simulink model "damped_non_linear"  (R2019a)
settings: Solver=VariableStepAuto  StartTime=0.0  StopTime=10.0  RelTol=1e-3
settings Model: Creator=iyengar  LastModifiedBy=iyengar

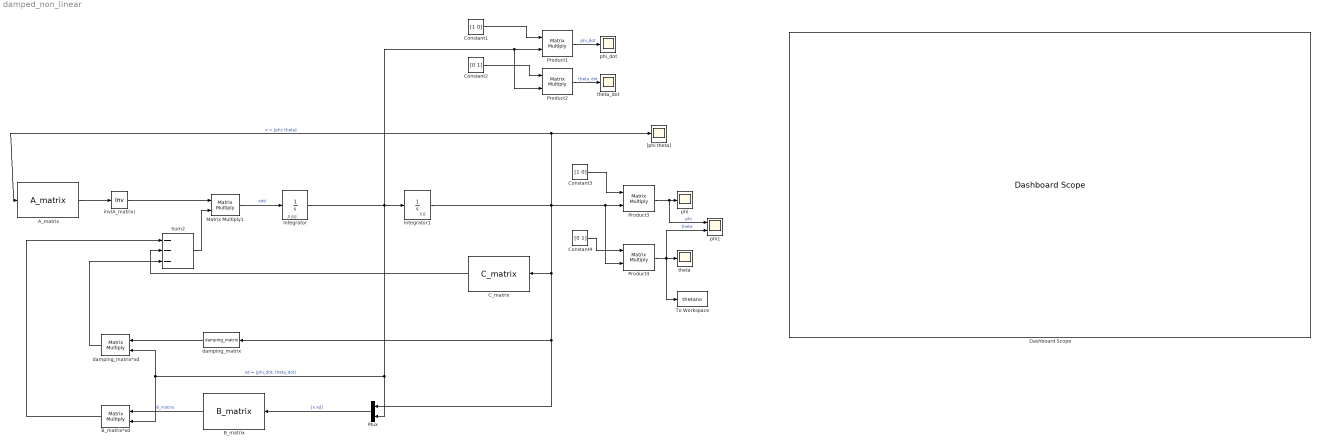
== system damped_non_linear ==
  note: Xdd
  note: Xd
  "A_matrix " : MATLABFcn  Description=matrix A. 2x2  MATLABFcn=A_matrix  OutputDimensions=[2, 2]  Output1D=off
  B_matrix : MATLABFcn  MATLABFcn=B_matrix  Output1D=off
  B_matrix*xd : Product  Multiplication=Matrix(*)
  C_matrix : MATLABFcn  MATLABFcn=C_matrix  OutputDimensions=2  Output1D=off
  Constant1 : Constant  Value=[1 0]  VectorParams1D=off
  Constant2 : Constant  Value=[0 1]  VectorParams1D=off
  Constant3 : Constant  Value=[1 0]  VectorParams1D=off
  Constant4 : Constant  Value=[0 1]  VectorParams1D=off
  Dashboard Scope : DashboardScope
  Integrator : Integrator  InitialCondition=[0; 0.5]
  Integrator1 : Integrator  InitialCondition=[0; 0.05]
  Matrix Multiply1 : Product  Multiplication=Matrix(*)
  Mux : Mux  Inputs=2
  Product{1..4} (4 alike) : Product  Multiplication=Matrix(*)
  Sum2 : Sum  Inputs=---
  To Workspace : ToWorkspace  VariableName=thetano  SaveFormat=Timeseries  SampleTime=-1
  "[phi theta]" : Scope
  damping_matrix : MATLABFcn  MATLABFcn=damping_matrix  Output1D=off
  "damping_matrix*xd " : Product  Multiplication=Matrix(*)
  inv(A_matrix) : Product  Inputs=/  Multiplication=Matrix(*)
  phi : Scope
  phi1 : Scope  NumInputPorts=2
  phi_dot : Scope
  theta : Scope
  theta_dot : Scope
  wires:
  B_matrix*xd/1 -> Sum2/1
  Sum2/1 -> Matrix Multiply1/2
  Constant4/1 -> Product4/1
  Matrix Multiply1/1 -> Integrator/1  "xdd"
  Product2/1 -> theta_dot/1  "theta_dot"
  Product3/1 -> phi1/1, phi/1  "phi"
  B_matrix/1 -> B_matrix*xd/1  "B_matrix"
  Constant3/1 -> Product3/1
  Product4/1 -> To Workspace/1, phi1/2, theta/1  "theta"
  Mux/1 -> B_matrix/1  "[x xd]"
  inv(A_matrix)/1 -> Matrix Multiply1/1
  Integrator1/1 -> "A_matrix "/1, "[phi theta]"/1, damping_matrix/1, Mux/1, C_matrix/1, Product4/2, Product3/2  "x = [phi; theta]"
  Integrator/1 -> Product2/2, Product1/2, Integrator1/1, Mux/2, "damping_matrix*xd "/2, B_matrix*xd/2  "xd = [phi_dot; theta_dot]"
  Constant1/1 -> Product1/1
  Product1/1 -> phi_dot/1  "phi_dot"
  C_matrix/1 -> Sum2/2
  Constant2/1 -> Product2/1
  "A_matrix "/1 -> inv(A_matrix)/1
  damping_matrix/1 -> "damping_matrix*xd "/1
  "damping_matrix*xd "/1 -> Sum2/3
